simulink model "ClassSimulink"  (R2016b)
settings: Solver=ode45  StartTime=0.0  StopTime=100  RelTol=1e-3  EnableMultiTasking=on
undefined symbols (not defined in the file or in its folder): gfprimfd
libraries: commchan3 x4, commblkcod2 x4, commdigbbndam3 x4, commsink2 x3, commrandsrc2 x2, commutil2 x2, dspquant2 x2
settings Model: Creator=mohammadezaz  LastModifiedBy=ASUS
settings DataIOCC: LimitDataPoints=on  SaveFormat=Array
settings OptimizationCC: LifeSpan=inf
settings DebuggingCC: SolverPrmCheckMsg=warning  SFUnexpectedBacktrackingDiag=warning  SFNoUnconditionalDefaultTransitionDiag=warning  SFExecutionAtInitializationDiag=none
settings HardwareCC: ProdBitPerPointer=32  ProdBitPerSizeT=32  ProdBitPerPtrDiffT=32  ProdLargestAtomicFloat=None  ProdIntDivRoundTo=Undefined  ProdEndianess=Unspecified  ProdWordSize=32  ProdHWDeviceType=32-bit Generic
settings ModelReferenceCC: PropagateSignalLabelsOutOfModel=off
settings GRTTargetCC: TargetLangStandard=C89/C90 (ANSI)  GeneratePreprocessorConditionals=Disable all
settings ConfigComp: CovMetricSettings=dw  CovHtmlReporting=on  CovSaveCumulativeToWorkspaceVar=on  CovSaveSingleToWorkspaceVar=on  CovExternalEMLEnable=off  CovSFcnEnable=off

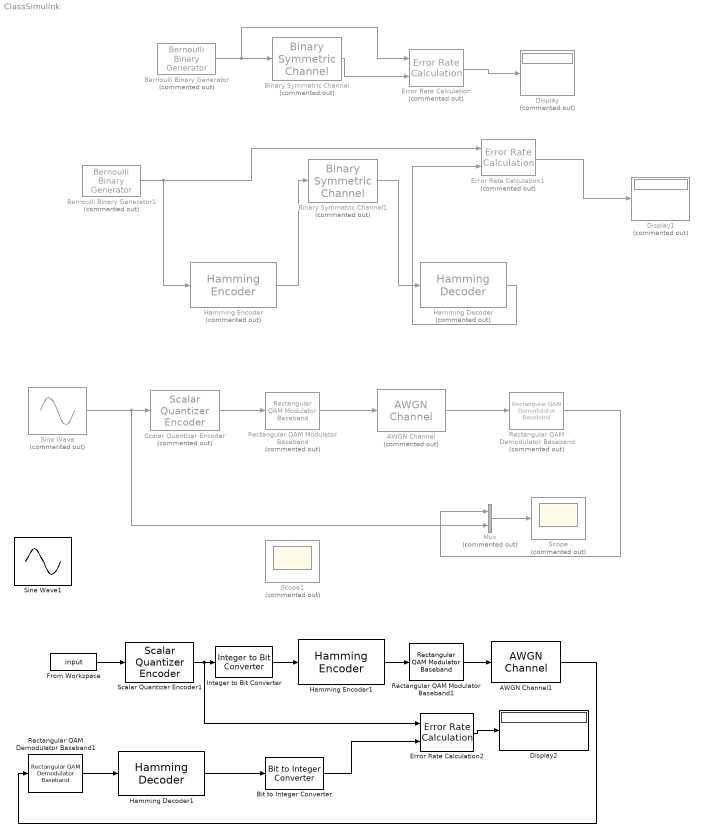
== system ClassSimulink ==
  AWGN Channel : commchan3/AWGN Channel  Commented=on  InputProcessing=Columns as channels (frame based)  seed=67  noiseMode="Signal to noise ratio  (Eb/No)"  EbNodB=20  EsNodB=10  SNRdB=10  bitsPerSym=1  Ps=1  Tsym=1  variance=1
  AWGN Channel1 : commchan3/AWGN Channel  InputProcessing=Columns as channels (frame based)  seed=67  noiseMode="Signal to noise ratio  (Eb/No)"  EbNodB=10  EsNodB=10  SNRdB=10  bitsPerSym=1  Ps=1  Tsym=1  variance=1
  Bernoulli Binary Generator : commrandsrc2/Bernoulli Binary Generator  Commented=on  P=0.5  seed=61  Ts=1  frameBased=off  sampPerFrame=1  orient=off  outDataType=double
  Bernoulli Binary Generator1 : commrandsrc2/Bernoulli Binary Generator  Commented=on  P=0.5  seed=61  Ts=1  frameBased=on  sampPerFrame=4  orient=off  outDataType=double
  Binary Symmetric Channel : commchan3/Binary Symmetric Channel  Commented=on  P=0.3  s=71  E=off  outDtype=double
  Binary Symmetric Channel1 : commchan3/Binary Symmetric Channel  Commented=on  P=0.3  s=71  E=off  outDtype=double
  Bit to Integer Converter : commutil2/Bit to Integer Converter  nbits=4  bitOrder=MSB first  signedOutputValues=Unsigned  outDtype=Inherit via internal rule  outDtypeSigned=Inherit via internal rule
  Display : Display  Commented=on
  Display1 : Display  Commented=on
  Display2 : Display
  Error Rate Calculation : commsink2/Error Rate Calculation  Commented=on  N=0  st_delay=0  cp_mode=Entire frame  subframe=[]  PMode=Port  WsName=ErrorVec  RsMode2=off  stop=off  numErr=100  maxBits=1e6
  Error Rate Calculation1 : commsink2/Error Rate Calculation  Commented=on  N=0  st_delay=0  cp_mode=Entire frame  subframe=[]  PMode=Port  WsName=ErrorVec  RsMode2=off  stop=off  numErr=100  maxBits=1e6
  Error Rate Calculation2 : commsink2/Error Rate Calculation  N=0  st_delay=0  cp_mode=Entire frame  subframe=[]  PMode=Port  WsName=ErrorVec  RsMode2=off  stop=off  numErr=100  maxBits=1e6
  From Workspace : FromWorkspace  VariableName=input  SampleTime=1
  Hamming Decoder : commblkcod2/Hamming Decoder  Commented=on  n=7  k=gfprimfd(3,'min')
  Hamming Decoder1 : commblkcod2/Hamming Decoder  n=7  k=gfprimfd(3,'min')
  Hamming Encoder : commblkcod2/Hamming Encoder  Commented=on  n=7  k=gfprimfd(3,'min')
  Hamming Encoder1 : commblkcod2/Hamming Encoder  n=7  k=gfprimfd(3,'min')
  Integer to Bit Converter : commutil2/Integer to Bit Converter  nbits=4  signedInputValues=Unsigned  bitOrder=MSB first  outDtype=Inherit via internal rule
  Mux : Mux  Commented=on  Inputs=2
  Rectangular QAM Demodulator Baseband : commdigbbndam3/Rectangular QAM Demodulator Baseband  Commented=on  M=16  OutType=Integer  DecType=Hard decision  VarSource=Dialog  Variance=1  Dec=Gray  Mapping=[0:15]  PowType=Min. distance between symbols  MinDist=2  AvgPow=1  PeakPow=1  Ph=0  outDtype1=Inherit via internal rule  outDtype2=Inherit via internal rule  derotateFactorWordLen=16  derotateFactorDataTypeStr=Inherit: Same word length as input  derotateFactorLastDataTypeStr=Inherit: Same word length as input  denormFactorWordLen=16  denormFactorDataTypeStr=Inherit: Same word length as input  denormFactorLastDataTypeStr=Inherit: Same word length as input  prodOutWordLen=32  prodOutOverflowMode=Wrap  prodOutRoundingMode=Floor  prodOutOvFlMode=off  prodOutOvFlModeLastStrValue=off  sumWordLen=32
  Rectangular QAM Demodulator Baseband1 : commdigbbndam3/Rectangular QAM Demodulator Baseband  M=128  OutType=Integer  DecType=Hard decision  VarSource=Dialog  Variance=1  Dec=Gray  Mapping=[0:15]  PowType=Min. distance between symbols  MinDist=2  AvgPow=1  PeakPow=1  Ph=0  outDtype1=Inherit via internal rule  outDtype2=Inherit via internal rule  derotateFactorWordLen=16  derotateFactorDataTypeStr=Inherit: Same word length as input  derotateFactorLastDataTypeStr=Inherit: Same word length as input  denormFactorWordLen=16  denormFactorDataTypeStr=Inherit: Same word length as input  denormFactorLastDataTypeStr=Inherit: Same word length as input  prodOutWordLen=32  prodOutOverflowMode=Wrap  prodOutRoundingMode=Floor  prodOutOvFlMode=off  prodOutOvFlModeLastStrValue=off  sumWordLen=32
  Rectangular QAM Modulator Baseband : commdigbbndam3/Rectangular QAM Modulator Baseband  Commented=on  M=16  InType=Integer  Enc=Gray  Mapping=[0:15]  PowType=Min. distance between symbols  MinDist=2  AvgPow=1  PeakPow=1  Ph=0  outDtype=double  outWordLen=16  outUDDataType=sfix(16)  outFracLenMode=Best precision  outFracLen=15  outDataTypeStr=double  outLastDataTypeStr=double
  Rectangular QAM Modulator Baseband1 : commdigbbndam3/Rectangular QAM Modulator Baseband  M=128  InType=Integer  Enc=Gray  Mapping=[0:15]  PowType=Min. distance between symbols  MinDist=2  AvgPow=1  PeakPow=1  Ph=0  outDtype=double  outWordLen=16  outUDDataType=sfix(16)  outFracLenMode=Best precision  outFracLen=15  outDataTypeStr=double  outLastDataTypeStr=double
  Scalar Quantizer Encoder : dspquant2/Scalar Quantizer Encoder  Commented=on  paramSrc=Specify via dialog  partType=Bounded  BBoundary=[-10:20/16:10]  UBoundary=[2:9]  SearchMethod=Linear  tieBreakRule=Choose the lower index  outQU=off  outQError=off  codebook=[1.5:9.5]  outStatus=off  invalidin=Clip  idtype=Inherit via back propagation  roundingMode=Floor  overflowMode=off
  Scalar Quantizer Encoder1 : dspquant2/Scalar Quantizer Encoder  paramSrc=Specify via dialog  partType=Bounded  BBoundary=[-10:20/16:10]  UBoundary=[2:9]  SearchMethod=Linear  tieBreakRule=Choose the lower index  outQU=off  outQError=off  codebook=[1.5:9.5]  outStatus=off  invalidin=Clip  idtype=int32  roundingMode=Floor  overflowMode=off
  Scope : Scope  Commented=on
  Scope1 : Scope  Commented=on
  Sine Wave : Sin  Commented=on  Amplitude=10  Frequency=10  SampleTime=0.001
  Sine Wave1 : Sin  Amplitude=10  Frequency=10  SampleTime=0.001
  wires:
  Bernoulli Binary Generator/1 -> Error Rate Calculation/1, Binary Symmetric Channel/1
  Binary Symmetric Channel/1 -> Error Rate Calculation/2
  Error Rate Calculation/1 -> Display/1
  Bernoulli Binary Generator1/1 -> Hamming Encoder/1, Error Rate Calculation1/1
  Error Rate Calculation1/1 -> Display1/1
  Hamming Encoder/1 -> Binary Symmetric Channel1/1
  Binary Symmetric Channel1/1 -> Hamming Decoder/1
  Hamming Decoder/1 -> Error Rate Calculation1/2
  Sine Wave/1 -> Mux/2, Scalar Quantizer Encoder/1
  Scalar Quantizer Encoder/1 -> Rectangular QAM Modulator Baseband/1
  Rectangular QAM Modulator Baseband/1 -> AWGN Channel/1
  AWGN Channel/1 -> Rectangular QAM Demodulator Baseband/1
  Rectangular QAM Demodulator Baseband/1 -> Mux/1
  Mux/1 -> Scope/1
  Scalar Quantizer Encoder1/1 -> Error Rate Calculation2/1, Integer to Bit Converter/1
  Integer to Bit Converter/1 -> Hamming Encoder1/1
  Hamming Encoder1/1 -> Rectangular QAM Modulator Baseband1/1
  Rectangular QAM Modulator Baseband1/1 -> AWGN Channel1/1
  AWGN Channel1/1 -> Rectangular QAM Demodulator Baseband1/1
  Rectangular QAM Demodulator Baseband1/1 -> Hamming Decoder1/1
  Hamming Decoder1/1 -> Bit to Integer Converter/1
  Error Rate Calculation2/1 -> Display2/1
  Bit to Integer Converter/1 -> Error Rate Calculation2/2
  From Workspace/1 -> Scalar Quantizer Encoder1/1
